simulink model "speed_control_disc_temporal_amplitud_delay"  (R2022b)
settings: Solver=VariableStepAuto  StartTime=0.0  StopTime=5  FixedStep=0.01  MaxStep=0.0005  RelTol=1e-3
libraries: simulink x4, slpidlib x2, autolibim x1, mcbplantlib x1, mcbcontrolslib x1
settings Model: Creator=mique  LastModifiedBy=mique
settings SolverCC: ZeroCrossAlgorithm=Adaptive
settings DebuggingCC: IgnoredZcDiagnostic=none

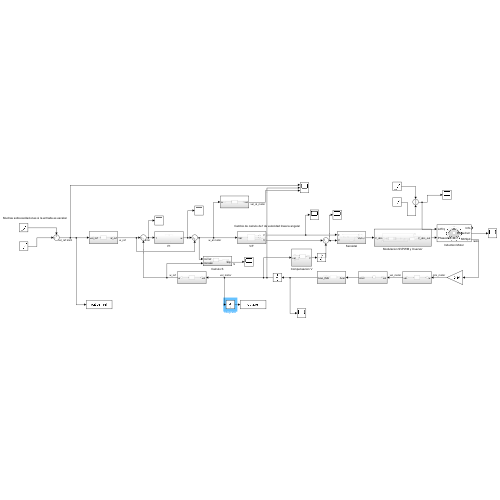
[thumbnail: Simulink's stored preview of the top-level diagram]
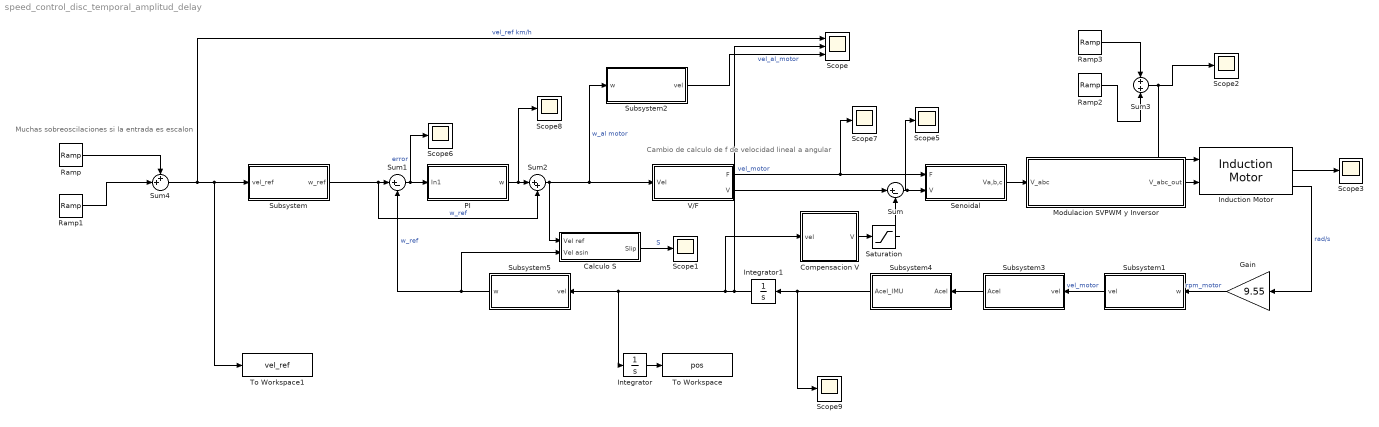
== system speed_control_disc_temporal_amplitud_delay ==
  note: Cambio de calculo de f de velocidad lineal a angular
  note: Muchas sobreoscilaciones si la entrada es escalon
  Calculo S : Subsystem
  Compensacion V : Subsystem
  Gain : Gain  Gain=9.55
  Induction Motor : autolibim/Induction Motor  sim_type=Continuous  Ts=0.001  port_config=Torque  P=8  Zs=[1.77 0.0139]  Zr="[1.34  0.0121]"  Lm=0.3687  mechanical=[0.01 0.059 0.01]  theta_init=0  omega_init=0  RefBlkName='autolibim/Induction Motor'  aMode=5
      settings: LibrarySourceBlock=mcblib/Electrical Systems/Motors/Induction Motor
  Integrator : Integrator
  Integrator1 : Integrator
  Modulacion SVPWM y Inversor : Subsystem
  PI : Subsystem
  Ramp : simulink/Sources/Ramp  slope=-70  start=0.5  InitialOutput=0
  Ramp1 : simulink/Sources/Ramp  slope=70  start=0  InitialOutput=0
  Ramp2 : simulink/Sources/Ramp  slope=0.5  start=0.1  InitialOutput=0
  Ramp3 : simulink/Sources/Ramp  slope=-0.5  start=5  InitialOutput=0
  Saturation : Saturate  UpperLimit=30  LowerLimit=0
  Scope : Scope  NumInputPorts=3
  Scope{1..3,5..9} (8 alike) : Scope
  Senoidal : Subsystem
  Subsystem : Subsystem
  Subsystem1 : Subsystem
  Subsystem2 : Subsystem
  Subsystem3 : Subsystem
  Subsystem4 : Subsystem
  Subsystem5 : Subsystem
  Sum : Sum  Inputs=|+-
  Sum1 : Sum  Inputs=|+-
  Sum2 : Sum  Inputs=|++
  Sum3 : Sum
  Sum4 : Sum  Inputs=++|
  To Workspace : ToWorkspace  VariableName=pos  SampleTime=-1
  To Workspace1 : ToWorkspace  VariableName=vel_ref  SampleTime=-1
  V/F : Subsystem
  wires:
  V/F/1(F) -> Scope7/1, Senoidal/1(F)
  Induction Motor/2 -> Scope3/1
  Senoidal/1(Va,b,c) -> Modulacion SVPWM y Inversor/1(V_abc)
  Induction Motor/3 -> Gain/1  "rad/s"
  Sum1/1 -> PI/1(In1), Scope6/1  "error"
  Sum3/1 -> Induction Motor/1, Scope2/1
  Modulacion SVPWM y Inversor/1(V_abc_out) -> Induction Motor/2
  Ramp3/1 -> Sum3/1
  Ramp2/1 -> Sum3/2
  Ramp1/1 -> Sum4/2
  Ramp/1 -> Sum4/1
  Sum4/1 -> To Workspace1/1, Subsystem/1(vel_ref), Scope/1  "vel_ref km/h"
  Subsystem2/1(vel) -> Scope/3  "vel_al_motor"
  Subsystem/1(w_ref) -> Sum2/2, Sum1/1  "w_ref"
  Sum2/1 -> V/F/1(Vel), Subsystem2/1(w), Calculo S/1(Vel ref)  "w_al motor"
  Calculo S/1(Slip) -> Scope1/1  "S"
  PI/1(w) -> Scope8/1, Sum2/1
  Sum/1 -> Scope5/1, Senoidal/2(V)
  V/F/2(V) -> Sum/1
  Compensacion V/1(V) -> Saturation/1
  Saturation/1 -> Sum/2
  Integrator/1 -> To Workspace/1
  Subsystem1/1(vel) -> Subsystem3/1(vel)  "vel_motor"
  Gain/1 -> Subsystem1/1(w)  "rpm_motor"
  Subsystem3/1(Acel) -> Subsystem4/1(Acel)
  Subsystem4/1(Acel_IMU) -> Integrator1/1, Scope9/1
  Integrator1/1 -> Integrator/1, Subsystem5/1(vel), Compensacion V/1(vel), Scope/2  "vel_motor"
  Subsystem5/1(w) -> Sum1/2, Calculo S/2(Vel asin)  "w_ref"

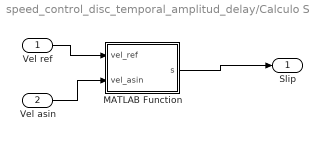
== system speed_control_disc_temporal_amplitud_delay/Calculo S ==
  Vel ref : Inport
  Vel asin : Inport  Port=2
  MATLAB Function : MATLAB Function  TreatAsAtomicUnit=on
  Slip : Outport
  wires:
  Vel ref/1 -> MATLAB Function/1(vel_ref)
  Vel asin/1 -> MATLAB Function/2(vel_asin)
  MATLAB Function/1(s) -> Slip/1

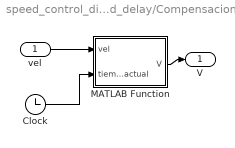
== system speed_control_disc_temporal_amplitud_delay/Compensacion V ==
  vel : Inport
  Clock : Clock
  MATLAB Function : MATLAB Function  TreatAsAtomicUnit=on
  V : Outport
  wires:
  vel/1 -> MATLAB Function/1(vel)
  MATLAB Function/1(V) -> V/1
  Clock/1 -> MATLAB Function/2(tiempo_actual)

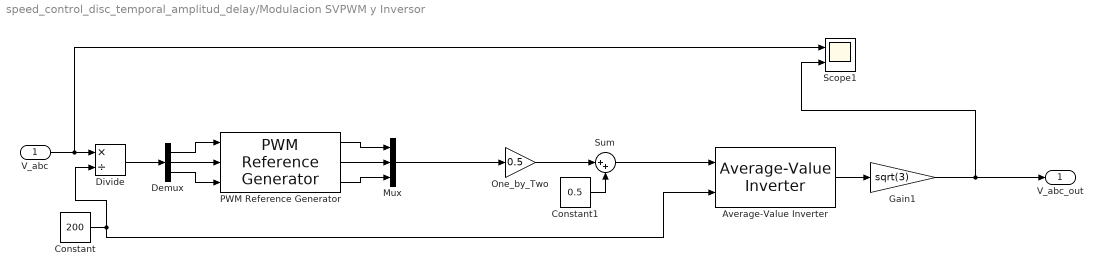
== system speed_control_disc_temporal_amplitud_delay/Modulacion SVPWM y Inversor ==
  V_abc : Inport
  Average-Value Inverter : mcbplantlib/Average-Value Inverter
      settings: LibrarySourceBlock=mcblib/Electrical Systems/Inverters/Average-Value Inverter
  Constant : Constant  Value=200
  Constant1 : Constant  Value=0.5  SampleTime=-1
  Demux : Demux  Outputs=3
  Divide : Product  Inputs=*/
  Gain1 : Gain  Gain=sqrt(3)
  Mux : Mux  Inputs=3
  One_by_Two : Gain  Gain=0.5  RndMeth=Simplest  OutDataTypeStr=Inherit: Same as input
  PWM Reference Generator : mcbcontrolslib/PWM Reference Generator  inSignal=Vabc  modType=SVM: space vector modulation
      settings: LibrarySourceBlock=mcbhdllib/Controls/Math Transforms/PWM Reference Generator
  Scope1 : Scope  NumInputPorts=2
  Sum : Sum  Inputs=|++
  V_abc_out : Outport
  wires:
  V_abc/1 -> Scope1/1, Divide/1
  PWM Reference Generator/1 -> Mux/1
  Demux/3 -> PWM Reference Generator/3
  Gain1/1 -> V_abc_out/1, Scope1/2
  Mux/1 -> One_by_Two/1
  PWM Reference Generator/2 -> Mux/2
  Constant/1 -> Divide/2, Average-Value Inverter/2
  Sum/1 -> Average-Value Inverter/1
  Demux/2 -> PWM Reference Generator/2
  PWM Reference Generator/3 -> Mux/3
  Demux/1 -> PWM Reference Generator/1
  One_by_Two/1 -> Sum/1
  Constant1/1 -> Sum/2
  Divide/1 -> Demux/1
  Average-Value Inverter/1 -> Gain1/1

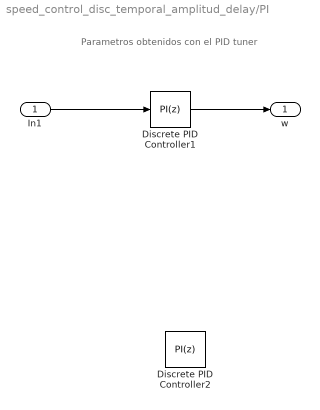
== system speed_control_disc_temporal_amplitud_delay/PI ==
  note: Parametros obtenidos con el PID tuner
  In1 : Inport
  Discrete PID Controller1 : slpidlib/PID Controller  Controller=PI  Form=Parallel  TimeDomain=Discrete-time  UseExternalTs=off  SampleTime=0.0005  IntegratorMethod=Forward Euler  FilterMethod=Forward Euler  ControllerParametersSource=internal  P=0.5  I=5  UseKiTs=off  D=0.0001  N=10  UseFilter=on  TunerSelectOption=Transfer Function Based (PID Tuner App)  InitialConditionSource=internal  InitialConditionForIntegrator=0  InitialConditionForFilter=0  DifferentiatorICPrevScaledInput=0  ExternalReset=none  TrackingMode=off  Kt=1  LimitOutput=off  SatLimitsSource=internal  UpperSaturationLimit=inf  LowerSaturationLimit=-inf  LinearizeAsGain=off  AntiWindupMode=back-calculation  Kb=1  LimitIntegrator=off  UpperIntegratorSaturationLimit=15  LowerIntegratorSaturationLimit=-15  POutMin=[]  POutMax=[]  IOutMin=[]  IOutMax=[]  DOutMin=[]  DOutMax=[]  NOutMin=[]  NOutMax=[]  SumOutMin=[]  SumOutMax=[]  SaturationOutMin=[]  SaturationOutMax=[]  PParamMin=[]  PParamMax=[]  IParamMin=[]  IParamMax=[]  DParamMin=[]  DParamMax=[]  NParamMin=[]  NParamMax=[]  KbParamMin=[]  KbParamMax=[]  KtParamMin=[]  KtParamMax=[]  KbOutMin=[]  KbOutMax=[]  KtOutMin=[]  KtOutMax=[]  IntegratorOutMin=[]  IntegratorOutMax=[]  FilterOutMin=[]  FilterOutMax=[]  SumI1OutMin=[]  SumI1OutMax=[]  SumI2OutMin=[]  SumI2OutMax=[]  SumI3OutMin=[]  SumI3OutMax=[]  SumI4OutMin=[]  SumI4OutMax=[]  SumDOutMin=[]  SumDOutMax=[]  DifferentiatorOutMin=[]  DifferentiatorOutMax=[]  FilterDiffOutCoefMin=[]  FilterDiffOutCoefMax=[]  ReciprocalOutMin=[]  ReciprocalOutMax=[]  SumDenOutMin=[]  SumDenOutMax=[]  SumNumOutMin=[]  SumNumOutMax=[]  DivideOutMin=[]  DivideOutMax=[]  UdiffTsProdOutMin=[]  UdiffTsProdOutMax=[]  NTsProdOutMin=[]  NTsProdOutMax=[]  UintegralTsProdOutMin=[]  UintegralTsProdOutMax=[]  UngainTsProdOutMin=[]  UngainTsProdOutMax=[]  ClampingZeroOutDataTypeStr=Inherit: Inherit via back propagation  ClampingZeroOutMin=[]  ClampingZeroOutMax=[]  FilterDenConstantOutDataTypeStr=Inherit: Inherit via back propagation  FilterDenConstantOutMin=[]  FilterDenConstantOutMax=[]  PCopyOutDataTypeStr=Inherit: Inherit via back propagation  PCopyOutMin=[]  PCopyOutMax=[]  NCopyOutDataTypeStr=Inherit: Inherit via back propagation  NCopyOutMin=[]  NCopyOutMax=[]  IntegratorContinuousStateAttributes=''  IntegratorStateMustResolveToSignalObject=off  IntegratorRTWStateStorageClass=Auto  FilterContinuousStateAttributes=''  FilterStateMustResolveToSignalObject=off  FilterRTWStateStorageClass=Auto  ParallelPVariant=InternalParameters  IdealPVariant=Disabled  IVariant=InternalParameters  DVariant=Disabled  IntegratorVariant=Discrete  SatVariant=Disabled  AWVariant=Passthrough  PCopyVariant=Disabled  TRVariant=Disabled  FdbkBlocksVariant=Forward  IdealPFdbkVariant=Disabled  SatFdbkVariant=Disabled  DerivativeFilterVariant=Disabled  NVariant=Disabled  NCopyVariant=Disabled_SignalSpec  FilterICVariant=Disabled  IntegratorICVariant=InternalICs  ExternalResetVariant=Disabled  TRSumVariant=Passthrough  SumFdbkVariant=Disabled  SumVariant=Sum_PI  TsampFilterVariant=InternalTs  TsampNgainVariant=Passthrough  TsampIntegralVariant=Passthrough  ExternalSaturationOutDataTypeStr=Inherit: Same as second input
      settings: LibrarySourceBlock=simulink/Discrete/Discrete PID Controller
  Discrete PID Controller2 : slpidlib/PID Controller  Controller=PI  Form=Parallel  TimeDomain=Discrete-time  UseExternalTs=off  SampleTime=0.0005  IntegratorMethod=Forward Euler  FilterMethod=Forward Euler  ControllerParametersSource=internal  P=1  I=8  UseKiTs=off  D=0.0001  N=10  UseFilter=on  TunerSelectOption=Transfer Function Based (PID Tuner App)  InitialConditionSource=internal  InitialConditionForIntegrator=0  InitialConditionForFilter=0  DifferentiatorICPrevScaledInput=0  ExternalReset=none  TrackingMode=off  Kt=1  LimitOutput=off  SatLimitsSource=internal  UpperSaturationLimit=inf  LowerSaturationLimit=-inf  LinearizeAsGain=off  AntiWindupMode=back-calculation  Kb=1  LimitIntegrator=off  UpperIntegratorSaturationLimit=15  LowerIntegratorSaturationLimit=-15  POutMin=[]  POutMax=[]  IOutMin=[]  IOutMax=[]  DOutMin=[]  DOutMax=[]  NOutMin=[]  NOutMax=[]  SumOutMin=[]  SumOutMax=[]  SaturationOutMin=[]  SaturationOutMax=[]  PParamMin=[]  PParamMax=[]  IParamMin=[]  IParamMax=[]  DParamMin=[]  DParamMax=[]  NParamMin=[]  NParamMax=[]  KbParamMin=[]  KbParamMax=[]  KtParamMin=[]  KtParamMax=[]  KbOutMin=[]  KbOutMax=[]  KtOutMin=[]  KtOutMax=[]  IntegratorOutMin=[]  IntegratorOutMax=[]  FilterOutMin=[]  FilterOutMax=[]  SumI1OutMin=[]  SumI1OutMax=[]  SumI2OutMin=[]  SumI2OutMax=[]  SumI3OutMin=[]  SumI3OutMax=[]  SumI4OutMin=[]  SumI4OutMax=[]  SumDOutMin=[]  SumDOutMax=[]  DifferentiatorOutMin=[]  DifferentiatorOutMax=[]  FilterDiffOutCoefMin=[]  FilterDiffOutCoefMax=[]  ReciprocalOutMin=[]  ReciprocalOutMax=[]  SumDenOutMin=[]  SumDenOutMax=[]  SumNumOutMin=[]  SumNumOutMax=[]  DivideOutMin=[]  DivideOutMax=[]  UdiffTsProdOutMin=[]  UdiffTsProdOutMax=[]  NTsProdOutMin=[]  NTsProdOutMax=[]  UintegralTsProdOutMin=[]  UintegralTsProdOutMax=[]  UngainTsProdOutMin=[]  UngainTsProdOutMax=[]  ClampingZeroOutDataTypeStr=Inherit: Inherit via back propagation  ClampingZeroOutMin=[]  ClampingZeroOutMax=[]  FilterDenConstantOutDataTypeStr=Inherit: Inherit via back propagation  FilterDenConstantOutMin=[]  FilterDenConstantOutMax=[]  PCopyOutDataTypeStr=Inherit: Inherit via back propagation  PCopyOutMin=[]  PCopyOutMax=[]  NCopyOutDataTypeStr=Inherit: Inherit via back propagation  NCopyOutMin=[]  NCopyOutMax=[]  IntegratorContinuousStateAttributes=''  IntegratorStateMustResolveToSignalObject=off  IntegratorRTWStateStorageClass=Auto  FilterContinuousStateAttributes=''  FilterStateMustResolveToSignalObject=off  FilterRTWStateStorageClass=Auto  ParallelPVariant=InternalParameters  IdealPVariant=Disabled  IVariant=InternalParameters  DVariant=Disabled  IntegratorVariant=Discrete  SatVariant=Disabled  AWVariant=Passthrough  PCopyVariant=Disabled  TRVariant=Disabled  FdbkBlocksVariant=Forward  IdealPFdbkVariant=Disabled  SatFdbkVariant=Disabled  DerivativeFilterVariant=Disabled  NVariant=Disabled  NCopyVariant=Disabled_SignalSpec  FilterICVariant=Disabled  IntegratorICVariant=InternalICs  ExternalResetVariant=Disabled  TRSumVariant=Passthrough  SumFdbkVariant=Disabled  SumVariant=Sum_PI  TsampFilterVariant=InternalTs  TsampNgainVariant=Passthrough  TsampIntegralVariant=Passthrough  ExternalSaturationOutDataTypeStr=Inherit: Same as second input
      settings: LibrarySourceBlock=simulink/Discrete/Discrete PID Controller
  w : Outport
  wires:
  In1/1 -> Discrete PID Controller1/1
  Discrete PID Controller1/1 -> w/1

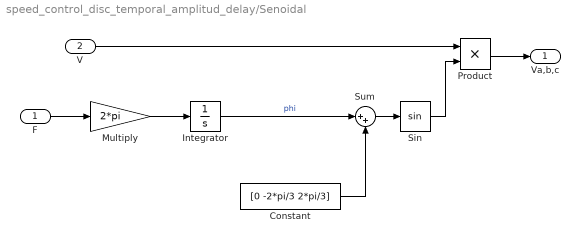
== system speed_control_disc_temporal_amplitud_delay/Senoidal ==
  F : Inport
  V : Inport  Port=2
  Constant : Constant  Value=[0 -2*pi/3 2*pi/3]
  Integrator : Integrator  WrapState=on
  Multiply : Gain  Gain=2*pi
  Product : Product
  Sin : Trigonometry
  Sum : Sum  Inputs=|++
  Va,b,c : Outport
  wires:
  Integrator/1 -> Sum/1  "phi"
  Constant/1 -> Sum/2
  Sum/1 -> Sin/1
  V/1 -> Product/1
  Sin/1 -> Product/2
  Product/1 -> Va,b,c/1
  F/1 -> Multiply/1
  Multiply/1 -> Integrator/1

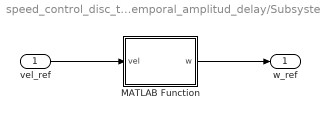
== system speed_control_disc_temporal_amplitud_delay/Subsystem ==
  vel_ref : Inport
  MATLAB Function : MATLAB Function  TreatAsAtomicUnit=on
  w_ref : Outport
  wires:
  vel_ref/1 -> MATLAB Function/1(vel)
  MATLAB Function/1(w) -> w_ref/1

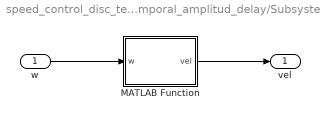
== system speed_control_disc_temporal_amplitud_delay/Subsystem1 ==
  w : Inport
  MATLAB Function : MATLAB Function  TreatAsAtomicUnit=on
  vel : Outport
  wires:
  w/1 -> MATLAB Function/1(w)
  MATLAB Function/1(vel) -> vel/1

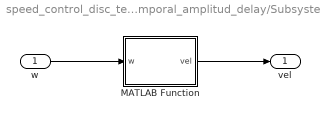
== system speed_control_disc_temporal_amplitud_delay/Subsystem2 ==
  w : Inport
  MATLAB Function : MATLAB Function  TreatAsAtomicUnit=on
  vel : Outport
  wires:
  w/1 -> MATLAB Function/1(w)
  MATLAB Function/1(vel) -> vel/1

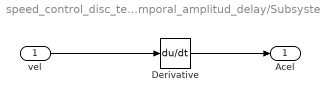
== system speed_control_disc_temporal_amplitud_delay/Subsystem3 ==
  vel : Inport
  Derivative : Derivative
  Acel : Outport
  wires:
  vel/1 -> Derivative/1
  Derivative/1 -> Acel/1

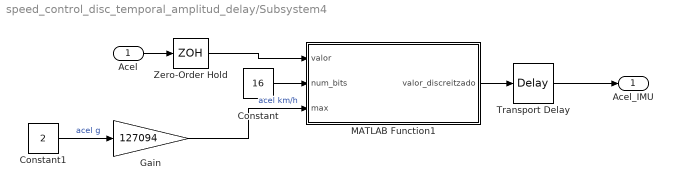
== system speed_control_disc_temporal_amplitud_delay/Subsystem4 ==
  Acel : Inport
  Constant : Constant  Value=16
  Constant1 : Constant  Value=2
  Gain : Gain  Gain=127094
  MATLAB Function1 : MATLAB Function  TreatAsAtomicUnit=on
  Transport Delay : TransportDelay  DelayTime=0.001
  Zero-Order Hold : ZeroOrderHold  SampleTime=0.0005
  Acel_IMU : Outport
  wires:
  Acel/1 -> Zero-Order Hold/1
  MATLAB Function1/1(valor_discreitzado) -> Transport Delay/1
  Zero-Order Hold/1 -> MATLAB Function1/1(valor)
  Constant1/1 -> Gain/1  "acel g"
  Constant/1 -> MATLAB Function1/2(num_bits)
  Gain/1 -> MATLAB Function1/3(max)  "acel km/h"
  Transport Delay/1 -> Acel_IMU/1

== system speed_control_disc_temporal_amplitud_delay/Subsystem5 ==
  vel : Inport
  MATLAB Function : MATLAB Function  TreatAsAtomicUnit=on
  w : Outport
  wires:
  MATLAB Function/1(w) -> w/1
  vel/1 -> MATLAB Function/1(vel)

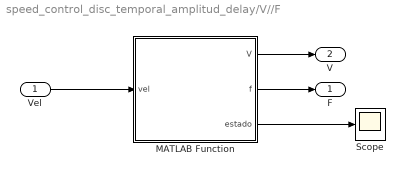
== system speed_control_disc_temporal_amplitud_delay/V//F ==
  Vel : Inport
  MATLAB Function : MATLAB Function  TreatAsAtomicUnit=on
  Scope : Scope
  F : Outport
  V : Outport  Port=2
  wires:
  Vel/1 -> MATLAB Function/1(vel)
  MATLAB Function/1(V) -> V/1
  MATLAB Function/2(f) -> F/1
  MATLAB Function/3(estado) -> Scope/1

== matlab function speed_control_disc_temporal_amplitud_delay/Subsystem/MATLAB Function ==
  data: vel input; w output
function w = fcn(vel)

num_parejas_Polos=8;

%Paso polar en metros
paso_polar=0.114;

%De km/h a m/s
vel_m=vel/3.6;

distancia_angular_parejas_polos=2*pi/(num_parejas_Polos*2);

%Velocidad en rad/s
w=vel_m*distancia_angular_parejas_polos/paso_polar;

%Velocidad en rpm
w=w*9.54;

== matlab function speed_control_disc_temporal_amplitud_delay/V//F/MATLAB Function ==
  data: vel input; V output; f output; estado output
function [V,f,estado]= v_f(vel)
estado=0;
num_parejas_Polos=8;

%Velocidad en RPM
f=vel*num_parejas_Polos/60;

if(f==0)
    f=0.0001;
    V=0;
    return
end

%F en HZ

%Comprobar valores
f_corte_inf=4;
V_min=15;
V_max=200;
f_corte_sup=f_corte_inf*V_max/V_min;

if(f<f_corte_inf)
    V=V_min;
    estado=0;
elseif(f<f_corte_sup)
    V=V_min/f_corte_inf*f;
    estado=1;
else
    V=V_max;
    estado=2;
end

== matlab function speed_control_disc_temporal_amplitud_delay/Subsystem1/MATLAB Function ==
  data: w input; vel output
function vel = fcn(w)

%Paso polar en metros
paso_polar=0.114;

num_parejas_Polos=8;

distancia_angular_parejas_polos=2*pi/(num_parejas_Polos*2);

%De rpm a rad/s
w=w/9.54;

vel_m=w*paso_polar/distancia_angular_parejas_polos;

%De m/s a km/h
vel=vel_m*3.6;

== matlab function speed_control_disc_temporal_amplitud_delay/Subsystem2/MATLAB Function ==
  data: w input; vel output
function vel = fcn(w)

%Paso polar en metros
paso_polar=0.114;

num_parejas_Polos=8;

distancia_angular_parejas_polos=2*pi/(num_parejas_Polos*2);

%De rpm a rad/s
w=w/9.54;

vel_m=w*paso_polar/distancia_angular_parejas_polos;

%De m/s a km/h
vel=vel_m*3.6;

== matlab function speed_control_disc_temporal_amplitud_delay/Calculo S/MATLAB Function ==
  data: vel_ref input; s output; vel_asin input
function s = fcn(vel_ref,vel_asin)

if(vel_ref==0)
    s=0;
else
   s=(vel_ref-vel_asin)/vel_ref;

end

== matlab function speed_control_disc_temporal_amplitud_delay/Compensacion V/MATLAB Function ==
  settings: updateMethod=DISCRETE
  data: vel input; V output; tiempo_actual input
function V= fcn(vel,tiempo_actual)

%Inicializacion Variables
persistent V_aux
if isempty(V_aux)
        V_aux = 0;
end

persistent T_aux
if isempty(T_aux)
        T_aux = 0;
end

persistent iniciado
if isempty(iniciado)
        iniciado=false;
end

persistent regimen_permanente
if isempty(regimen_permanente)
        regimen_permanente=false;
end


%Esperando al transitorio
if(iniciado==false) 
    %Si estamos en permanente, se espera 0.5 segundo y si seguimos iniciamos
    %la reducción de voltaje
    if(vel>34.95)
        if(regimen_permanente==false)
            T_aux=tiempo_actual;
            regimen_permanente=true;
        end

        if(tiempo_actual>T_aux+0.5)
            iniciado=true;
        end
    else
        %No afectar al par en aceleración
        V_aux=0;
    end
end

if(iniciado)
    if(vel>34.95)
        %Velocidad cercana final->Buscar eficiencia
        if(tiempo_actual>T_aux+0.004)
            V_aux=V_aux+0.1;
            T_aux=tiempo_actual;
        end
    else
        %Velocidad cercana final disminuye->Buscar par
        if(tiempo_actual>T_aux+0.001)
            V_aux=V_aux-0.1;
            if(V_aux<0)
                V_aux=0;
            end
            T_aux=tiempo_actual;
        end
    end
end

V=V_aux;
end

== matlab function speed_control_disc_temporal_amplitud_delay/Subsystem5/MATLAB Function ==
  data: vel input; w output
function w = fcn(vel)

num_parejas_Polos=8;

%Paso polar en metros
paso_polar=0.114;

%De km/h a m/s
vel_m=vel/3.6;

distancia_angular_parejas_polos=2*pi/(num_parejas_Polos*2);

%Velocidad en rad/s
w=vel_m*distancia_angular_parejas_polos/paso_polar;

%Velocidad en rpm
w=w*9.54;

== matlab function speed_control_disc_temporal_amplitud_delay/Subsystem4/MATLAB Function1 ==
  data: valor input; valor_discreitzado output; num_bits input; max input
function valor_discreitzado  = fcn(valor,num_bits,max)

min=-max;
num_valores=2^num_bits;
if(valor>max)
    valor_discreitzado=max;
    return
end
if(valor<min)
    valor_discreitzado=min;
    return
end


valor_escalon=(max-min)/(num_valores-1);


i=min;
 while(i<max)
    if(i+valor_escalon/2>valor)
        valor_discreitzado=i;
        return
    end
    i=i+valor_escalon;
end



      valor_discreitzado=max;
end
